simulink model "Circuit2_v4"  (R2020b)
settings: Solver=ode4  StartTime=0.0  StopTime=5  FixedStep=1e-4  RelTol=1e-3
values from neighbouring files (symbols this model uses):
  A_spol = 1/4 * pi * Dspool^2    (= 7.85398163397e-05)    [Circuit2_values.m]
  Be = 1300e6    (= 1300000000)    [Circuit1_load.m]    (also in Circuit2_values.m)
  BeA = 1200e6    (= 1200000000)    [Circuit2_values.m]    (also in Circut3_values.m = 1300000000)
  BeB = 1500e6    (= 1500000000)    [Circuit2_values.m]    (also in Circut3_values.m = 1300000000)
  Cd = 0.7    [Circuit1_load.m]    (also in Circuit2_values.m)
  Dorifice = 2e-2    (= 0.02)    [Circuit1_load.m]    (also in Circuit2_values.m = 0.004)
  Kp = (1.e-3)/(10e5)    (= 1e-09)    [Circuit1_load.m]    (also in Circuit2_values.m; Circut3_values.m)
  pA0 = 1e5    (= 100000)    [Circuit2_values.m]    (also in Circut3_values.m = 7300000)
  pB0 = 1e5    (= 100000)    [Circuit2_values.m]    (also in Circut3_values.m = 700000)
  pp0 = 180e5    (= 18000000)    [Circuit2_values.m]
  pref = 180e5    (= 18000000)    [Circuit1_load.m]    (also in Circuit2_values.m; Circut3_values.m = 17000000)
  rho = 860    [Circuit1_load.m]    (also in Circuit2_values.m; Circut3_values.m)
  tau = 60e-3    (= 0.06)    [Circuit1_load.m]    (also in Circuit2_values.m = 0.03)
  V = 3e-3    (= 0.003)    [Circuit1_load.m]    (also in Circuit2_values.m)
  VA = 5e-4    (= 0.0005)    [Circuit2_values.m]    (also in Circut3_values.m = 0.0015)
  VB = 5e-4    (= 0.0005)    [Circuit2_values.m]    (also in Circut3_values.m = 0.003)
settings Model: Creator=Janne  LastModifiedBy=Alex
settings DataIOCC: ReturnWorkspaceOutputs=off
settings DebuggingCC: ArithmeticOperatorsInVariantConditions=warning
settings SFSimCC: CustomCodeUndefinedFunction=UseInterfaceOnly

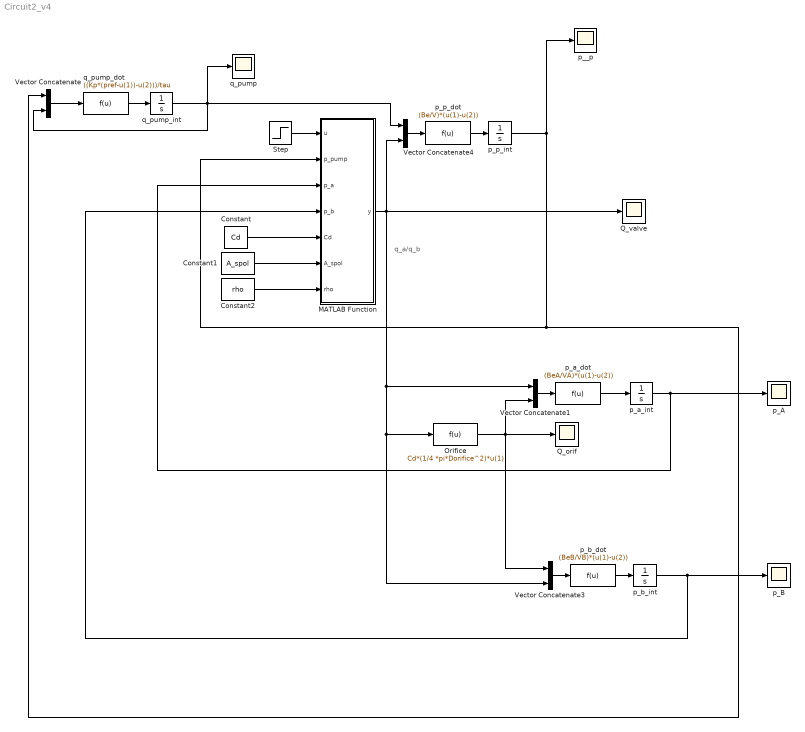
== system Circuit2_v4 ==
  note: q_a/q_b
  Constant : Constant  Value=Cd
  Constant1 : Constant  Value=A_spol
  Constant2 : Constant  Value=rho
  MATLAB Function : MATLAB Function  TreatAsAtomicUnit=on
  Orifice : Fcn  Expr=Cd*(1/4 *pi*Dorifice^2)*u(1)
  Q_orif : Scope
  Q_valve : Scope
  Step : Step  Time=2  Before=-0.0004  After=0.0004  SampleTime=0
  Vector Concatenate{,1,3..4} (4 alike) : Concatenate
  p_A : Scope
  p_B : Scope
  p__p : Scope
  p_a_dot : Fcn  Expr=(BeA/VA)*(u(1)-u(2))
  p_a_int : Integrator  InitialCondition=pA0  LimitOutput=on  UpperSaturationLimit=1000e5  LowerSaturationLimit=0
  p_b_dot : Fcn  Expr=(BeB/VB)*(u(1)-u(2))
  p_b_int : Integrator  InitialCondition=pB0  LimitOutput=on  UpperSaturationLimit=1000e5  LowerSaturationLimit=0
  p_p_dot : Fcn  Expr=(Be/V)*(u(1)-u(2))
  p_p_int : Integrator  InitialCondition=pp0  LimitOutput=on  UpperSaturationLimit=1000e5  LowerSaturationLimit=0
  q_pump : Scope
  q_pump_dot : Fcn  Expr=((Kp*(pref-u(1))-u(2)))/tau
  q_pump_int : Integrator  LimitOutput=on  UpperSaturationLimit=1000e5  LowerSaturationLimit=0
  wires:
  q_pump_dot/1 -> q_pump_int/1
  Vector Concatenate/1 -> q_pump_dot/1
  q_pump_int/1 -> q_pump/1, Vector Concatenate/2, Vector Concatenate4/1
  Vector Concatenate4/1 -> p_p_dot/1
  p_p_dot/1 -> p_p_int/1
  Step/1 -> MATLAB Function/1(u)
  p_p_int/1 -> Vector Concatenate/1, MATLAB Function/2(p_pump), p__p/1
  Constant/1 -> MATLAB Function/5(Cd)
  Constant1/1 -> MATLAB Function/6(A_spol)
  Constant2/1 -> MATLAB Function/7(rho)
  p_a_dot/1 -> p_a_int/1
  p_b_dot/1 -> p_b_int/1
  Vector Concatenate1/1 -> p_a_dot/1
  Vector Concatenate3/1 -> p_b_dot/1
  Orifice/1 -> Q_orif/1, Vector Concatenate3/1, Vector Concatenate1/2
  p_a_int/1 -> p_A/1, MATLAB Function/3(p_a)
  p_b_int/1 -> p_B/1, MATLAB Function/4(p_b)
  MATLAB Function/1(y) -> Vector Concatenate1/1, Vector Concatenate3/2, Orifice/1, Q_valve/1, Vector Concatenate4/2

== matlab function Circuit2_v4/MATLAB Function ==
  data: u input; p_pump input; p_a input; p_b input; y output; Cd input; A_spol input; rho input
function y = fcn(u, p_pump, p_a, p_b, Cd, A_spol, rho)
 q_PA = Cd*A_spol * abs(u) *sqrt(2*abs(p_pump-p_a)/rho);
 q_PB = Cd*A_spol * abs(u) *sqrt(2*abs(p_pump-p_b)/rho);
 
 if u >= 0
     q_out = q_PA;
 else
     q_out = -q_PB;
 end
y = q_out;
